simulink model "BaseEngineController_LS_128"  (Simulink 7.7)
settings: Solver=FixedStepDiscrete  StartTime=0.0  StopTime=10.0  RelTol=1e-3
PreLoadFcn:
  | try, eval([bdroot '_setup']); catch, eval('model_setup', ''); end
InitFcn:
  | try, eval([bdroot '_setup']); catch, eval('model_setup', ''); end
undefined symbols (not defined in the file): ECU565, High, motohawk_build_version, motohawk_trunc_name, motohawk_vardec_config_group, motohawk_vardec_path, True
libraries: MotoHawk_lib x1418, motohawk_control_primitives_lib x183, motohawk_engine_lib x32, simulink x21, motohawk_annotations_lib x9, AutoDoc_lib x8, simulink_extras x4, motohawk_ccp_examples_lib x1, motohawk_control_primitives_motoshare_lib x1
(part 27 of 27)

== system BaseEngineController_LS_128/Foreground/Control/Diagnostics/MISFIRE/MisfireDiagSub/MisfireDiagFunc/DetermineMisfire/SetHardFault ==
  CylNum : Inport
  Compare To Constant : simulink/Logic and Bit Operations/Compare To Constant  SystemSampleTime=-1  relop===  const=1  LogicOutDataTypeMode=boolean
  Compare To Constant1 : simulink/Logic and Bit Operations/Compare To Constant  SystemSampleTime=-1  relop===  const=2  LogicOutDataTypeMode=boolean
  Compare To Constant2 : simulink/Logic and Bit Operations/Compare To Constant  SystemSampleTime=-1  relop===  const=3  LogicOutDataTypeMode=boolean
  Compare To Constant3 : simulink/Logic and Bit Operations/Compare To Constant  SystemSampleTime=-1  relop===  const=4  LogicOutDataTypeMode=boolean
  Compare To Constant4 : simulink/Logic and Bit Operations/Compare To Constant  SystemSampleTime=-1  relop===  const=5  LogicOutDataTypeMode=boolean
  Compare To Constant5 : simulink/Logic and Bit Operations/Compare To Constant  SystemSampleTime=-1  relop===  const=6  LogicOutDataTypeMode=boolean
  Compare To Constant6 : simulink/Logic and Bit Operations/Compare To Constant  SystemSampleTime=-1  relop===  const=7  LogicOutDataTypeMode=boolean
  Compare To Constant7 : simulink/Logic and Bit Operations/Compare To Constant  SystemSampleTime=-1  relop===  const=8  LogicOutDataTypeMode=boolean
  motohawk_fault_def : MotoHawk_lib/Fault Management Blocks/motohawk_fault_def  nam='Cylinder1_HardMisfire'  mode=Enabled  id=[]  x=25  y=50  input_suspected=on  indeterminate=off  increment_xy=on  downsample_count=1  ovr_cals=on  ovr_actions=on  show_actions=off  action1_name=''  action1_cond=(None)  action2_name=''  action2_cond=(None)  action3_name=''  action3_cond=(None)  action4_name=''  action4_cond=(None)
  motohawk_fault_def1 : MotoHawk_lib/Fault Management Blocks/motohawk_fault_def  nam='Cylinder2_HardMisfire'  mode=Enabled  id=[]  x=25  y=50  input_suspected=on  indeterminate=off  increment_xy=on  downsample_count=1  ovr_cals=on  ovr_actions=on  show_actions=off  action1_name=''  action1_cond=(None)  action2_name=''  action2_cond=(None)  action3_name=''  action3_cond=(None)  action4_name=''  action4_cond=(None)
  motohawk_fault_def2 : MotoHawk_lib/Fault Management Blocks/motohawk_fault_def  nam='Cylinder3_HardMisfire'  mode=Enabled  id=[]  x=25  y=50  input_suspected=on  indeterminate=off  increment_xy=on  downsample_count=1  ovr_cals=on  ovr_actions=on  show_actions=off  action1_name=''  action1_cond=(None)  action2_name=''  action2_cond=(None)  action3_name=''  action3_cond=(None)  action4_name=''  action4_cond=(None)
  motohawk_fault_def3 : MotoHawk_lib/Fault Management Blocks/motohawk_fault_def  nam='Cylinder4_HardMisfire'  mode=Enabled  id=[]  x=25  y=50  input_suspected=on  indeterminate=off  increment_xy=on  downsample_count=1  ovr_cals=on  ovr_actions=on  show_actions=off  action1_name=''  action1_cond=(None)  action2_name=''  action2_cond=(None)  action3_name=''  action3_cond=(None)  action4_name=''  action4_cond=(None)
  motohawk_fault_def4 : MotoHawk_lib/Fault Management Blocks/motohawk_fault_def  nam='Cylinder5_HardMisfire'  mode=Enabled  id=[]  x=25  y=50  input_suspected=on  indeterminate=off  increment_xy=on  downsample_count=1  ovr_cals=on  ovr_actions=on  show_actions=off  action1_name=''  action1_cond=(None)  action2_name=''  action2_cond=(None)  action3_name=''  action3_cond=(None)  action4_name=''  action4_cond=(None)
  motohawk_fault_def5 : MotoHawk_lib/Fault Management Blocks/motohawk_fault_def  nam='Cylinder6_HardMisfire'  mode=Enabled  id=[]  x=25  y=50  input_suspected=on  indeterminate=off  increment_xy=on  downsample_count=1  ovr_cals=on  ovr_actions=on  show_actions=off  action1_name=''  action1_cond=(None)  action2_name=''  action2_cond=(None)  action3_name=''  action3_cond=(None)  action4_name=''  action4_cond=(None)
  motohawk_fault_def6 : MotoHawk_lib/Fault Management Blocks/motohawk_fault_def  nam='Cylinder7_HardMisfire'  mode=Enabled  id=[]  x=25  y=50  input_suspected=on  indeterminate=off  increment_xy=on  downsample_count=1  ovr_cals=on  ovr_actions=on  show_actions=off  action1_name=''  action1_cond=(None)  action2_name=''  action2_cond=(None)  action3_name=''  action3_cond=(None)  action4_name=''  action4_cond=(None)
  motohawk_fault_def7 : MotoHawk_lib/Fault Management Blocks/motohawk_fault_def  nam='Cylinder8_HardMisfire'  mode=Enabled  id=[]  x=25  y=50  input_suspected=on  indeterminate=off  increment_xy=on  downsample_count=1  ovr_cals=on  ovr_actions=on  show_actions=off  action1_name=''  action1_cond=(None)  action2_name=''  action2_cond=(None)  action3_name=''  action3_cond=(None)  action4_name=''  action4_cond=(None)
  wires:
  CylNum/1 -> Compare To Constant/1, Compare To Constant1/1, Compare To Constant2/1, Compare To Constant3/1, Compare To Constant4/1, Compare To Constant5/1, Compare To Constant6/1, Compare To Constant7/1
  Compare To Constant/1 -> motohawk_fault_def/1
  Compare To Constant7/1 -> motohawk_fault_def7/1
  Compare To Constant6/1 -> motohawk_fault_def6/1
  Compare To Constant5/1 -> motohawk_fault_def5/1
  Compare To Constant4/1 -> motohawk_fault_def4/1
  Compare To Constant3/1 -> motohawk_fault_def3/1
  Compare To Constant2/1 -> motohawk_fault_def2/1
  Compare To Constant1/1 -> motohawk_fault_def1/1

== system BaseEngineController_LS_128/Foreground/Control/Diagnostics/MISFIRE/MisfireDiagSub/MisfireDiagFunc/StoreRPMData/DetermineCylinder ==
  ArrayIn : Inport
  Constant : Constant  Value=[1,2,3,4,5,6,7,8]
  MinMax : MinMax  Function=max
  Product : Product  RndMeth=Zero
  CylinderNum : Outport
  wires:
  ArrayIn/1 -> Product/1
  Constant/1 -> Product/2
  Product/1 -> MinMax/1
  MinMax/1 -> CylinderNum/1

== system BaseEngineController_LS_128/Foreground/Control/Diagnostics/MISFIRE/MisfireDiagSub/MisfireDiagFunc/StoreRPMData/DetermineCylinder1 ==
  ArrayIn : Inport
  Constant : Constant  Value=[1,2,3,4,5,6,7,8]
  MinMax : MinMax  Function=max
  Product : Product  RndMeth=Zero
  CylinderNum : Outport
  wires:
  ArrayIn/1 -> Product/1
  Constant/1 -> Product/2
  Product/1 -> MinMax/1
  MinMax/1 -> CylinderNum/1

== system BaseEngineController_LS_128/Foreground/Control/Diagnostics/MISFIRE/MisfireDiagSub/MisfireDiagFunc/StoreRPMData/EncoderAngleArb ==
  Data Type Conversion : DataTypeConversion  OutDataTypeStr=int16
  EncoderAngle_wExtrap : Subsystem  TreatAsAtomicUnit=on
  EncoderAngle_wOExtrap : Subsystem  TreatAsAtomicUnit=on
  If : If  IfExpression=u1 ~= 0
  Merge : Merge
  motohawk_calibration3 : MotoHawk_lib/Calibration & Probing Blocks/motohawk_calibration  nam='MisfireDiag_EncoderExtrap_MPC5XX'  val=0  storage=Calibration  show_more=on  name_source=Use Parameter  data_type=boolean  read_level=1  write_level=1  ovr_cals=on  view_as=Enumeration  enum_struct={'Disabled', 'Enabled'}  vector_style=Wide Row  use_help_units=off  help=''  units=''  use_header_enum=off  row_header_enum={}  col_header_enum={}  use_min_max=off  min_val=-inf  max_val=inf  use_precision=off  precision=''  gain=1  offset=0  exp=1  use_mototune_group=off  mototune_group=motohawk_vardec_path(gcb)
  EncoderAngle_116 : Outport
  wires:
  motohawk_calibration3/1 -> If/1
  EncoderAngle_wExtrap/1(EncoderAngle) -> Data Type Conversion/1
  EncoderAngle_wOExtrap/1(EncoderAngle) -> Merge/1
  Merge/1 -> EncoderAngle_116/1
  If/1 -> EncoderAngle_wExtrap/Action
  If/2 -> EncoderAngle_wOExtrap/Action
  Data Type Conversion/1 -> Merge/2

== system BaseEngineController_LS_128/Foreground/Control/Diagnostics/MISFIRE/MisfireDiagSub/MisfireDiagFunc/StoreRPMData/LatchForAverage ==
  Enbl : Inport
  Constant : Constant
  Constant1 : Constant  Value=0
  Constant3 : Constant  Value=0  OutDataTypeStr=uint16
  GetInstRPM : Subsystem  TreatAsAtomicUnit=on
  Relational Operator : RelationalOperator  OutDataTypeStr=boolean
  S-R Flip-Flop : simulink_extras/Flip Flops/S-R Flip-Flop  SystemSampleTime=-1  initial_condition=0
  SafeDivide : Subsystem  TreatAsAtomicUnit=on
  Sum : Sum  SaturateOnIntegerOverflow=on  InputSameDT=on  OutDataTypeStr=Inherit: Same as first input
  Sum1 : Sum  SaturateOnIntegerOverflow=on  InputSameDT=on  OutDataTypeStr=Inherit: Same as first input
  Switch : Switch  Threshold=0.5  SaturateOnIntegerOverflow=on  InputSameDT=on
  Switch1 : Switch  Threshold=0.5  OutDataTypeStr=uint16  SaturateOnIntegerOverflow=on  InputSameDT=on
  Terminator : Terminator
  Unit Delay1 : UnitDelay  SampleTime=-1
  Unit Delay2 : UnitDelay  SampleTime=-1
  motohawk_calibration : MotoHawk_lib/Calibration & Probing Blocks/motohawk_calibration  nam='MisfireDiag_StartRPMAvgCnt'  val=3  storage=Calibration  show_more=on  name_source=Use Parameter  data_type=uint8  read_level=1  write_level=1  ovr_cals=on  view_as=Number  enum_struct={'Disabled', 'Enabled'}  vector_style=Wide Row  use_help_units=off  help=''  units=''  use_header_enum=off  row_header_enum={}  col_header_enum={}  use_min_max=off  min_val=-inf  max_val=inf  use_precision=off  precision=''  gain=1  offset=0  exp=1  use_mototune_group=off  mototune_group=motohawk_vardec_path(gcb)
  AverageRPMDR : Outport
  AverageRPM : Outport  Port=2
  wires:
  Enbl/1 -> S-R Flip-Flop/1
  S-R Flip-Flop/2 -> Switch/2, Switch1/2, GetInstRPM/Enable
  motohawk_calibration/1 -> Relational Operator/2, SafeDivide/1(Count)
  Relational Operator/1 -> AverageRPMDR/1, [RPMAvgDR]
  Unit Delay2/1 -> Sum/2, Relational Operator/1
  Switch/1 -> Unit Delay2/1
  Constant1/1 -> Switch/1
  Sum/1 -> Switch/3
  Constant/1 -> Sum/1
  Unit Delay1/1 -> Sum1/2, SafeDivide/2(RPMSum)
  Switch1/1 -> Unit Delay1/1
  Constant3/1 -> Switch1/1
  Sum1/1 -> Switch1/3
  GetInstRPM/1(InstRPM) -> Sum1/1
  SafeDivide/1(RPMAvg) -> AverageRPM/1
  [RPMAvgDR] -> S-R Flip-Flop/2
  [RPMAvgDR] -> SafeDivide/Enable
  S-R Flip-Flop/1 -> Terminator/1

== system BaseEngineController_LS_128/Foreground/Control/Diagnostics/MISFIRE/MisfireDiagSub/MisfireDiagFunc/StoreRPMData/LatchForAverage1 ==
  Enbl : Inport
  Constant : Constant
  Constant1 : Constant  Value=0
  Constant3 : Constant  Value=0  OutDataTypeStr=uint16
  GetInstRPM : Subsystem  TreatAsAtomicUnit=on
  Relational Operator : RelationalOperator  OutDataTypeStr=boolean
  S-R Flip-Flop : simulink_extras/Flip Flops/S-R Flip-Flop  SystemSampleTime=-1  initial_condition=0
  SafeDivide : Subsystem  TreatAsAtomicUnit=on
  Sum : Sum  SaturateOnIntegerOverflow=on  InputSameDT=on  OutDataTypeStr=Inherit: Same as first input
  Sum1 : Sum  SaturateOnIntegerOverflow=on  InputSameDT=on  OutDataTypeStr=Inherit: Same as first input
  Switch : Switch  Threshold=0.5  SaturateOnIntegerOverflow=on  InputSameDT=on
  Switch1 : Switch  Threshold=0.5  OutDataTypeStr=uint16  SaturateOnIntegerOverflow=on  InputSameDT=on
  Terminator : Terminator
  Unit Delay1 : UnitDelay  SampleTime=-1
  Unit Delay2 : UnitDelay  SampleTime=-1
  motohawk_calibration : MotoHawk_lib/Calibration & Probing Blocks/motohawk_calibration  nam='MisfireDiag_StopRPMAvgCnt'  val=3  storage=Calibration  show_more=on  name_source=Use Parameter  data_type=uint8  read_level=1  write_level=1  ovr_cals=on  view_as=Number  enum_struct={'Disabled', 'Enabled'}  vector_style=Wide Row  use_help_units=off  help=''  units=''  use_header_enum=off  row_header_enum={}  col_header_enum={}  use_min_max=off  min_val=-inf  max_val=inf  use_precision=off  precision=''  gain=1  offset=0  exp=1  use_mototune_group=off  mototune_group=motohawk_vardec_path(gcb)
  AverageRPMDR : Outport
  AverageRPM : Outport  Port=2
  wires:
  Enbl/1 -> S-R Flip-Flop/1
  S-R Flip-Flop/2 -> Switch/2, Switch1/2, GetInstRPM/Enable
  motohawk_calibration/1 -> Relational Operator/2, SafeDivide/1(Count)
  Relational Operator/1 -> AverageRPMDR/1, [RPMAvgDR]
  Unit Delay2/1 -> Sum/2, Relational Operator/1
  Switch/1 -> Unit Delay2/1
  Constant1/1 -> Switch/1
  Sum/1 -> Switch/3
  Constant/1 -> Sum/1
  Unit Delay1/1 -> Sum1/2, SafeDivide/2(RPMSum)
  Switch1/1 -> Unit Delay1/1
  Constant3/1 -> Switch1/1
  Sum1/1 -> Switch1/3
  GetInstRPM/1(InstRPM) -> Sum1/1
  SafeDivide/1(RPMAvg) -> AverageRPM/1
  [RPMAvgDR] -> S-R Flip-Flop/2
  [RPMAvgDR] -> SafeDivide/Enable
  S-R Flip-Flop/1 -> Terminator/1

== system BaseEngineController_LS_128/Foreground/Control/Diagnostics/MISFIRE/MisfireDiagSub/MisfireDiagFunc/StoreRPMData/StoreRPMStart ==
  AverageRPM : Inport
  CylinderNum : Inport  Port=2
  Enable : EnablePort
  Constant : Constant  Value=0  OutDataTypeStr=boolean
  motohawk_data_write : MotoHawk_lib/Data Storage Blocks/motohawk_data_write  source=Lookup By Name  structure=Vector  operation=Write scalar into location by index  sz_vec=8  sz_row=2  sz_col=9  typ=uint16  nam='MisfireDiag_StartRPM'  checkNull=on  write_read_only=off  struct_inst_name=''  struct_name='MyStruct'
  motohawk_data_write1 : MotoHawk_lib/Data Storage Blocks/motohawk_data_write  source=Lookup By Name  structure=Vector  operation=Write scalar into location by index  sz_vec=8  sz_row=2  sz_col=9  typ=boolean  nam='MisfireDiag_RPMDR'  checkNull=on  write_read_only=off  struct_inst_name=''  struct_name='MyStruct'
  wires:
  AverageRPM/1 -> motohawk_data_write/1
  CylinderNum/1 -> motohawk_data_write/2, motohawk_data_write1/2
  Constant/1 -> motohawk_data_write1/1

== system BaseEngineController_LS_128/Foreground/Control/Diagnostics/MISFIRE/MisfireDiagSub/MisfireDiagFunc/StoreRPMData/StoreRPMStart1 ==
  AverageRPM : Inport
  CylinderNum : Inport  Port=2
  Enable : EnablePort
  Constant : Constant  OutDataTypeStr=boolean
  motohawk_data_write : MotoHawk_lib/Data Storage Blocks/motohawk_data_write  source=Lookup By Name  structure=Vector  operation=Write scalar into location by index  sz_vec=8  sz_row=2  sz_col=9  typ=uint16  nam='MisfireDiag_StopRPM'  checkNull=on  write_read_only=off  struct_inst_name=''  struct_name='MyStruct'
  motohawk_data_write1 : MotoHawk_lib/Data Storage Blocks/motohawk_data_write  source=Lookup By Name  structure=Vector  operation=Write scalar into location by index  sz_vec=8  sz_row=2  sz_col=9  typ=boolean  nam='MisfireDiag_RPMDR'  checkNull=on  write_read_only=off  struct_inst_name=''  struct_name='MyStruct'
  wires:
  Constant/1 -> motohawk_data_write1/1
  AverageRPM/1 -> motohawk_data_write/1
  CylinderNum/1 -> motohawk_data_write/2, motohawk_data_write1/2

== system BaseEngineController_LS_128/Foreground/Control/Diagnostics/MISFIRE/MisfireDiagSub/MisfireDiagFunc/StoreRPMData/EncoderAngleArb/EncoderAngle_wExtrap ==
  Action Port : ActionPort  ActionType=then
  motohawk_encoder_angle_extrapolation : MotoHawk_lib/Encoder Blocks/motohawk_encoder_angle_extrapolation  SystemSampleTime=-1  cdeg=16  group=motohawk_vardec_path(gcb)
  EncoderAngle : Outport
  wires:
  motohawk_encoder_angle_extrapolation/1 -> EncoderAngle/1

== system BaseEngineController_LS_128/Foreground/Control/Diagnostics/MISFIRE/MisfireDiagSub/MisfireDiagFunc/StoreRPMData/EncoderAngleArb/EncoderAngle_wOExtrap ==
  Action Port : ActionPort  ActionType=else
  motohawk_encoder_angle : MotoHawk_lib/Encoder Blocks/motohawk_encoder_angle
  EncoderAngle : Outport
  wires:
  motohawk_encoder_angle/1 -> EncoderAngle/1

== system BaseEngineController_LS_128/Foreground/Control/Diagnostics/MISFIRE/MisfireDiagSub/MisfireDiagFunc/StoreRPMData/LatchForAverage/GetInstRPM ==
  Enable : EnablePort
  motohawk_encoder_instant_rpm : MotoHawk_lib/Encoder Blocks/motohawk_encoder_instant_rpm
  InstRPM : Outport
  wires:
  motohawk_encoder_instant_rpm/1 -> InstRPM/1

== system BaseEngineController_LS_128/Foreground/Control/Diagnostics/MISFIRE/MisfireDiagSub/MisfireDiagFunc/StoreRPMData/LatchForAverage/SafeDivide ==
  Count : Inport
  RPMSum : Inport  Port=2
  Enable : EnablePort
  Constant : Constant  OutDataTypeStr=uint16
  MinMax : MinMax  Function=max  Inputs=2
  Product : Product  Inputs=*/  OutDataTypeStr=uint16  RndMeth=Zero
  RPMAvg : Outport
  wires:
  RPMSum/1 -> Product/1
  Product/1 -> RPMAvg/1
  Count/1 -> MinMax/1
  MinMax/1 -> Product/2
  Constant/1 -> MinMax/2

== system BaseEngineController_LS_128/Foreground/Control/Diagnostics/MISFIRE/MisfireDiagSub/MisfireDiagFunc/StoreRPMData/LatchForAverage1/GetInstRPM ==
  Enable : EnablePort
  motohawk_encoder_instant_rpm : MotoHawk_lib/Encoder Blocks/motohawk_encoder_instant_rpm
  InstRPM : Outport
  wires:
  motohawk_encoder_instant_rpm/1 -> InstRPM/1

== system BaseEngineController_LS_128/Foreground/Control/Diagnostics/MISFIRE/MisfireDiagSub/MisfireDiagFunc/StoreRPMData/LatchForAverage1/SafeDivide ==
  Count : Inport
  RPMSum : Inport  Port=2
  Enable : EnablePort
  Constant : Constant  OutDataTypeStr=uint16
  MinMax : MinMax  Function=max  Inputs=2
  Product : Product  Inputs=*/  OutDataTypeStr=uint16  RndMeth=Zero
  RPMAvg : Outport
  wires:
  RPMSum/1 -> Product/1
  Product/1 -> RPMAvg/1
  Count/1 -> MinMax/1
  MinMax/1 -> Product/2
  Constant/1 -> MinMax/2

== stateflow chart Foreground/Control/VirtualSensors/RawProcessed/EngineState/Engine State Machine ==
  settings: executeAtInitialization=1
  state Stall/
    en:State=1;
  state Run/
    en:State=3;
  state Crank/
    en:State=2;
  (default) -> Stall
  Stall -> Crank : [Crank]
  Crank -> Run [order 2] : [Run]
  Run -> Stall : [Stall]
  Crank -> Stall [order 1] : [Stall]
  data: Stall input boolean; Crank input boolean; Run input boolean; State output uint8

== stateflow chart Foreground/Control/Controller/Stall/Stall Throttle/Ice Break ==
  state Init
    du:
    etc = 0;
  state Open
    du:
    etc = icePos;
  state Wait
    du:
    etc = 0;
  (default) -> Init
  Init -> Open : [timeSinceKeyOn < enblTime]
  Open -> Wait : after(hldTime,sec)
  Wait -> Init : [timeSinceKeyOn > enblTime]
  data: etc output double; timeSinceKeyOn input double; enblTime input double; hldTime input double; icePos input double

== matlab function Foreground/Control/Controller/Run/MaxGovernor/MaxGovState/MaxGOV Stateflow ==
  data: OffToOn input double; ETCMode output double; OnToTrans input double; TransToOn input double; TransToOff input double; State input double; Reset output double; Hold output double; StateO output double
function [ETCMode,Reset,Hold,StateO] = fcn(OffToOn,OnToTrans,TransToOn,TransToOff,State)

if (State == 0 && OffToOn == 1)
    StateO = 1;
elseif (State == 1 && OnToTrans == 1)
    StateO=2;
elseif (State == 2 && TransToOn == 1)
    StateO=1;
elseif (State == 2 && TransToOff == 1)
    StateO=0;
else
    StateO=State;
end

if State == 0
    ETCMode=0;
    Hold=0;
    Reset=0;
elseif State == 1;
    ETCMode=1;
    Hold=0;
    Reset=0;
elseif State == 2;
    ETCMode=0;
    Hold=1;
    Reset=0;
else
    ETCMode=0;
    Hold=0;
    Reset=0;
end

== stateflow chart Main Power Relay/Main Power Relay/ECUP Latch ==
  settings: executeAtInitialization=1
  state PowerDown/
    en:MPRDState=0;
  state PowerUp/
    en:MPRDState=1;
  (default) -> PowerDown
  PowerUp -> PowerDown : [!ECUP&&ShutDownTasks]
  PowerDown -> PowerUp : [ECUP]
  data: ECUP input boolean; ShutDownTasks input boolean; MPRDState output boolean

== stateflow chart Foreground/Control/ActuatorCharacterization/Electronic Throttle Controller/ETC Test  Manager ==
  settings: executeAtInitialization=1
  state PassThrough/
    en:DC_Override=0;
    en:TestComplete=0;
    en:SetpointMode=0;
    en:TestTime=0;
  state LowAdapt/
    en:DC_Override=0;
    en:TestComplete=0;
    en:SetpointMode=1;
    en:TestTime=0;
  state SpringTestSetpoint/
    en:DC_Override=0;
    en:TestComplete=0;
    en:SetpointMode=2;
    en:TestTime=0;
  state SpringTest/
    en:DC_Override=1;
    en:TestComplete=0;
    en:SetpointMode=0;
    en:TestTime=0;
    en:TimerOld=Timer;
  state SpringTestComplete/
    en:DC_Override=1;
    en:TestComplete=1;
    en:SetpointMode=0;
    en:TestTime=Timer-TimerOld;
  state ForcedShutdown/
    en:DC_Override=1;
    en:TestComplete=1;
    en:SetpointMode=0;
    en:TestTime=0;
  (default) -> PassThrough
  PassThrough -> LowAdapt : [ECUP_Off]
  LowAdapt -> SpringTestSetpoint [order 2] : [ECUP_Off&&LowAdaptError]
  SpringTestSetpoint -> SpringTest [order 2] : [ECUP_Off&&TPSHiThresh]
  SpringTest -> SpringTestComplete [order 2] : [ECUP_Off&&TPSLoThresh]
  LowAdapt -> PassThrough [order 3] : [!ECUP_Off]
  SpringTestSetpoint -> PassThrough [order 1] : [!ECUP_Off]
  SpringTestComplete -> PassThrough : [!ECUP_Off]
  SpringTest -> PassThrough [order 3] : [!ECUP_Off]
  SpringTest -> ForcedShutdown [order 1] : [Timer>5]
  LowAdapt -> ForcedShutdown [order 1] : [Timer>5]
  SpringTestSetpoint -> ForcedShutdown [order 3] : [Timer>5]
  ForcedShutdown -> SpringTestComplete : [!ECUP_Off]
  data: TestTime output double; ECUP_Off input boolean; DC_Override output int8; Timer input double; LowAdaptError input boolean; TPSHiThresh input boolean; TPSLoThresh input boolean; TimerOld local double; TestComplete output boolean; SetpointMode output int8

== matlab function Foreground/Outputs/Coil Control/Coil Enable Manager/EST Enable TDC Counter/EST Enable TDC Counter Stateflow ==
  data: CounterEnabled input double; CounterReset output double; EngineState input double; State input double; ESTEnable output double; StateO output double
function [CounterReset,ESTEnable,StateO] = fcn(CounterEnabled,EngineState,State)

if (State == 0 && CounterEnabled == 1)
    StateO=1;
elseif (State == 1 && EngineState == 2 && CounterEnabled == 1)
    StateO=2;
elseif (State == 2 && EngineState ==3)
    StateO=3;
elseif (State == 2 && EngineState == 1)
    StateO=0;
elseif (State ==3 && EngineState == 1)
    StateO=0;
else
    StateO=State;
end

if State == 0
   ESTEnable=0;
   CounterReset=0;
elseif State == 1
    ESTEnable=1;
    CounterReset=0;
elseif State == 2
    ESTEnable=1;
    CounterReset=1;
elseif State == 3
    ESTEnable=1;
    CounterReset=1;
else
    ESTEnable=0;
    CounterReset=0;
end

== stateflow chart Foreground/Control/Controller/Run/MinGovernor/Idle State Determination/IdleStateMachine ==
  state OffIdle/
    en:IdleState = 3;
  state Flaring/
    en:IdleState = 1;
  state OnIdle/
    en:IdleState = 2;
  (default) -> Flaring
  Flaring -> OffIdle [order 1] : [ThrCmdHigh || !IdleEnable]
  OffIdle -> OnIdle : [IdleEnable && (RPMLow || (RPMInRange && ...
      | ThrCmdLow)) || APPTimeThresh]
  Flaring -> OnIdle [order 2] : [RPMFalling && ThrCmdLow]
  OnIdle -> OffIdle : [!RPMLow&&(ThrCmdHigh || !IdleEnable)]
  data: IdleEnable input boolean; RPMFalling input boolean; RPMInRange input boolean; RPMLow input boolean; ThrCmdLow input boolean; ThrCmdHigh input boolean; IdleState output uint8; APPTimeThresh input boolean

== stateflow chart Foreground/Control/VirtualSensors/AirCalcs/Baro Stall State Delay ==
  settings: executeAtInitialization=1
  state Stall/
    en:Enable=1;
  state CrankRun/
    en:Enable=0;
  state StallDelay/
    en:Enable=0;
    en:Timer=0;
    en:TOld=0;
    during:Timer=TOld+dT;
    during:TOld=Timer;
  (default) -> Stall
  Stall -> CrankRun : [EngineState>1]
  CrankRun -> StallDelay : [EngineState==1]
  StallDelay -> Stall [order 2] : [EngineState==1&Timer>TimeThresh]
  StallDelay -> CrankRun [order 1] : [EngineState>1]
  data: EngineState input uint8; TimeThresh input double; dT input double; Timer output double; Enable output boolean; TOld local double
